simulink model "hemZ_PWMstudy_3level_23b"  (R2023b)
settings: Solver=FixedStepAuto  StartTime=0.0  StopTime=2e-3  FixedStep=1e-7  MaxStep=1e-7  RelTol=1e-3
libraries: spsTriangleGeneratorLib x4
settings Model: Creator=lbocker  LastModifiedBy=enesa
settings DebuggingCC: SignalInfNanChecking=warning

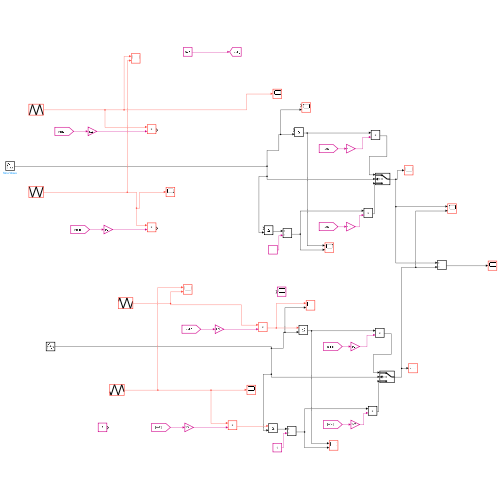
[thumbnail: Simulink's stored preview of the top-level diagram]
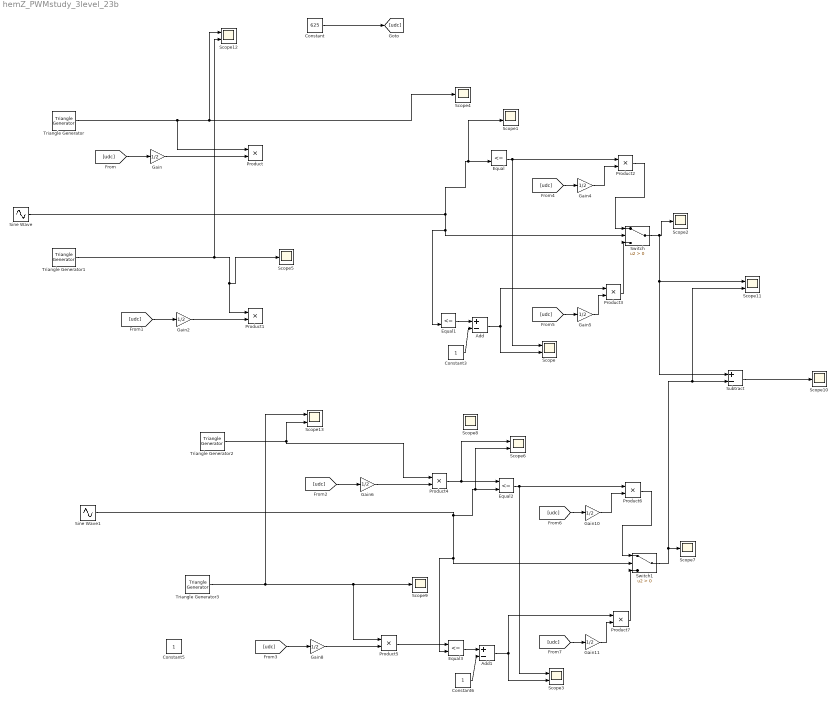
== system hemZ_PWMstudy_3level_23b ==
  Add : Sum  Inputs=+-
  Add1 : Sum  Inputs=+-
  Constant : Constant  Value=625
  Constant3 : Constant
  Constant5 : Constant
  Constant6 : Constant
  Equal{,1..3} (4 alike) : RelationalOperator  Operator=<=  OutDataTypeStr=boolean  RndMeth=Simplest  InputSameDT=off
  Gain{,2,4..6,8,10..11} (8 alike) : Gain  Gain=1/2
  Product{,1..7} (8 alike) : Product
  Scope{,1,3,6,11..13} (7 alike) : Scope  NumInputPorts=2
  Scope{2,4..5,7..10} (7 alike) : Scope
  Sine Wave : Sin  Amplitude=0.8*625/2  Frequency=2*pi*500  SampleTime=0
  Sine Wave1 : Sin  Amplitude=0.8*625/2  Frequency=2*pi*500  Phase=2*pi/3  SampleTime=0
  Subtract : Sum  Inputs=+-
  Switch : Switch  Criteria=u2 > Threshold  SaturateOnIntegerOverflow=off  InputSameDT=off
  Switch1 : Switch  Criteria=u2 > Threshold  SaturateOnIntegerOverflow=off  InputSameDT=off
  Triangle Generator : spsTriangleGeneratorLib/Triangle Generator  Freq=30e3  Phase=0  Ts=1e-7
  Triangle Generator1 : spsTriangleGeneratorLib/Triangle Generator  Freq=30e3  Phase=180  Ts=1e-7
  Triangle Generator2 : spsTriangleGeneratorLib/Triangle Generator  Freq=30e3  Phase=120  Ts=1e-7
  Triangle Generator3 : spsTriangleGeneratorLib/Triangle Generator  Freq=30e3  Phase=120+180  Ts=1e-7
  wires:
  Product3/1 -> Switch/3
  [udc] -> Gain5/1
  Gain4/1 -> Product2/2
  [udc] -> Gain4/1
  Add/1 -> Product3/1, Scope/2
  Constant3/1 -> Add/2
  Equal1/1 -> Add/1
  Sine Wave/1 -> Scope1/2, Equal/2, Switch/2, Equal1/2
  Gain5/1 -> Product3/2
  Gain2/1 -> Product1/2
  Constant/1 -> [udc]
  [udc] -> Gain/1
  Triangle Generator1/1 -> Scope12/2, Product1/1, Scope5/1
  Gain/1 -> Product/2
  Triangle Generator/1 -> Scope4/1, Scope12/1, Product/1
  [udc] -> Gain2/1
  Equal/1 -> Scope/1, Product2/1
  Product2/1 -> Switch/1
  [udc] -> Gain8/1
  Equal2/1 -> Scope3/1, Product6/1
  Gain8/1 -> Product5/2
  Gain11/1 -> Product7/2
  Product5/1 -> Equal3/1
  Gain6/1 -> Product4/2
  Product4/1 -> Scope6/1, Equal2/1
  Constant6/1 -> Add1/2
  Switch1/1 -> Scope11/2, Subtract/2, Scope7/1
  [udc] -> Gain10/1
  Gain10/1 -> Product6/2
  [udc] -> Gain11/1
  Product6/1 -> Switch1/1
  Add1/1 -> Product7/1, Scope3/2
  Product7/1 -> Switch1/3
  Equal3/1 -> Add1/1
  [udc] -> Gain6/1
  Sine Wave1/1 -> Switch1/2, Equal3/2, Scope6/2, Equal2/2
  Subtract/1 -> Scope10/1
  Switch/1 -> Subtract/1, Scope11/1, Scope2/1
  Triangle Generator2/1 -> Product4/1, Scope13/2
  Triangle Generator3/1 -> Scope13/1, Scope9/1, Product5/1
